simulink model "reflex"  (R2017b)
settings: Solver=VariableStepAuto  StartTime=0.0  StopTime=20  RelTol=1e-3
settings Model: Creator=Lenovo  LastModifiedBy=Lenovo

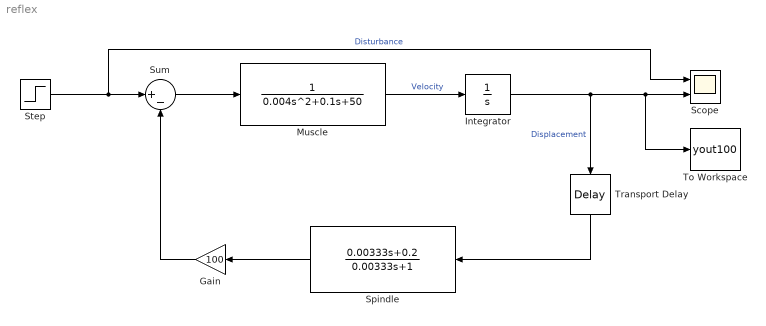
== system reflex ==
  Gain : Gain  Gain=100
  Integrator : Integrator
  Muscle : TransferFcn  Denominator=[0.004 0.1 50]
  Scope : Scope  NumInputPorts=2
  Spindle : TransferFcn  Numerator=[0.00333 0.2]  Denominator=[0.00333 1]
  Step : Step  Time=0  After=5  SampleTime=0
  Sum : Sum  Inputs=|+-
  To Workspace : ToWorkspace  VariableName=yout100  SampleTime=-1
      settings: Save2DSignal=2-D array (concatenate along first dimension)
  Transport Delay : TransportDelay  DelayTime=0.005
  wires:
  Sum/1 -> Muscle/1
  Muscle/1 -> Integrator/1  "Velocity"
  Spindle/1 -> Gain/1
  Gain/1 -> Sum/2
  Integrator/1 -> To Workspace/1, Scope/2, Transport Delay/1  "Displacement"
  Transport Delay/1 -> Spindle/1
  Step/1 -> Scope/1, Sum/1  "Disturbance"
